simulink model "SIM_continuousFermenter"  (R2023b)
settings: Solver=VariableStepAuto  StartTime=0.0  StopTime=500  RelTol=1e-3
values from neighbouring files (symbols this model uses):
  Ts = 0.5    [MHE_compute2.m]
libraries: mpclib x1, SignalEditorBlockLib x1
settings Model: Creator=akeebismail  LastModifiedBy=akeebismail

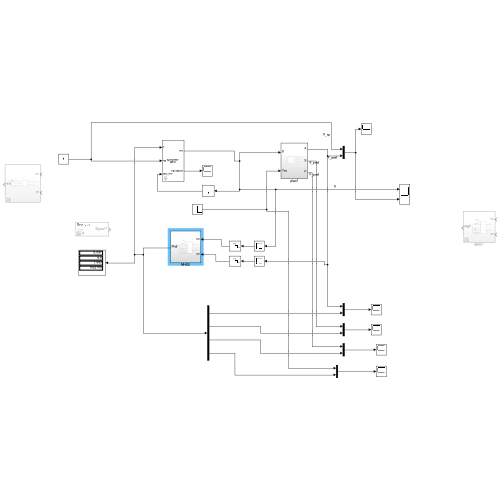
[thumbnail: Simulink's stored preview of the top-level diagram]
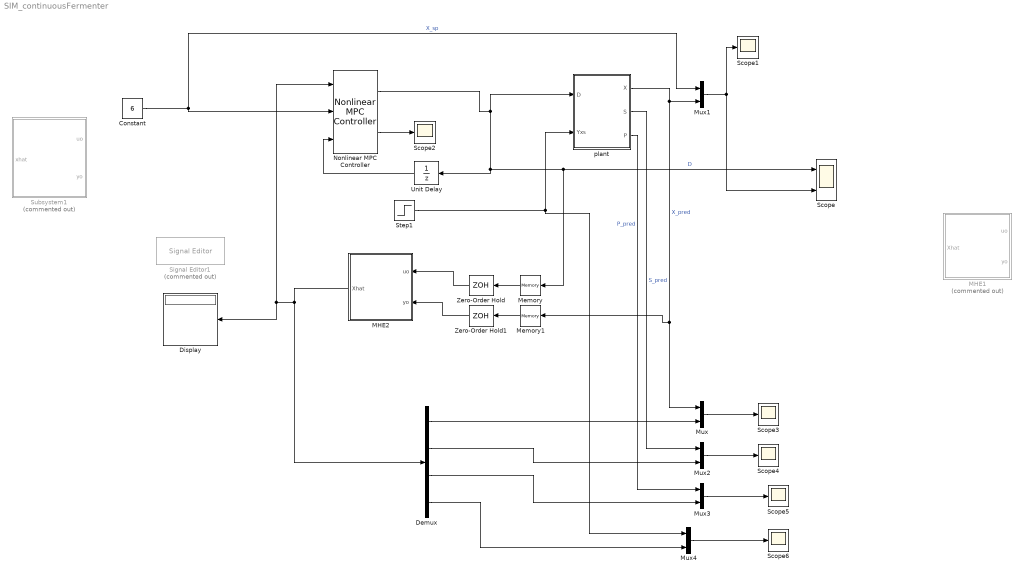
== system SIM_continuousFermenter ==
  Constant : Constant  Value=6
  Demux : Demux
  Display : Display
  MHE1 : Subsystem  Commented=on
  MHE2 : Subsystem
  Memory : Memory  InitialCondition=0.202
  Memory1 : Memory  InitialCondition=6
  Mux{,1..4} (5 alike) : Mux  Inputs=2
  Nonlinear MPC Controller : mpclib/Nonlinear MPC Controller  nlmpcobj=nlobj  UseObjectTs=on  UseMEX=off  md_enabled=off  mvtarget_enabled=off  param_enabled=off  cost_enabled=off  mvseq_enabled=off  stateseq_enabled=off  ovseq_enabled=off  slack_enabled=off  status_enabled=on  ov_min=off  ov_max=off  mv_min=off  mv_max=off  mvrate_min=off  mvrate_max=off  state_min=off  state_max=off  ov_weight=off  mv_weight=off  mvrate_weight=off  ecr_weight=off  nlp_initialize=off
  Scope : Scope  NumInputPorts=2
  Scope{1..6} (6 alike) : Scope
  Signal Editor1 : SignalEditorBlockLib/Signal Editor  Commented=on  FileName=Yxs.mat  ActiveScenario=Scenario  ActiveSignal=Signal 1  IsBus=off  OutputBusObjectStr=Bus: BusObject  SampleTime=Ts  Interpolate=off  ZeroCross=off  OutputAfterFinalValue=Setting to zero  Unit=inherit  PreserveSignalName=on  ApplySigPropsToAllScenarios=on  ApplySigPropsToAllSignals=off
  Step1 : Step  Time=200  Before=0.4  After=0.35  SampleTime=0
  Subsystem1 : Subsystem  Commented=on
  Unit Delay : UnitDelay  InitialCondition=0.202  SampleTime=Ts  HasFrameUpgradeWarning=on
  Zero-Order Hold : ZeroOrderHold  SampleTime=Ts
  Zero-Order Hold1 : ZeroOrderHold  SampleTime=Ts
  plant : Subsystem
  wires:
  Nonlinear MPC Controller/1 -> Memory/1, Scope/1, Unit Delay/1, plant/1(D)  "D"
  Constant/1 -> Nonlinear MPC Controller/2, Mux1/1  "X_sp"
  Nonlinear MPC Controller/2 -> Scope2/1
  plant/1(X) -> Mux/1, Memory1/1, Mux1/2  "X_pred"
  Unit Delay/1 -> Nonlinear MPC Controller/3
  Mux1/1 -> Scope/2, Scope1/1
  Zero-Order Hold/1 -> MHE2/1(uo)
  Zero-Order Hold1/1 -> MHE2/2(yo)
  Memory/1 -> Zero-Order Hold/1
  Memory1/1 -> Zero-Order Hold1/1
  MHE2/1(Xhat) -> Demux/1, Nonlinear MPC Controller/1, Display/1
  Demux/1 -> Mux/2
  Demux/2 -> Mux2/2
  Demux/3 -> Mux3/2
  Demux/4 -> Mux4/2
  plant/2(S) -> Mux2/1  "S_pred"
  plant/3(P) -> Mux3/1  "P_pred"
  Step1/1 -> Mux4/1, plant/2(Yxs)
  Mux/1 -> Scope3/1
  Mux2/1 -> Scope4/1
  Mux3/1 -> Scope5/1
  Mux4/1 -> Scope6/1

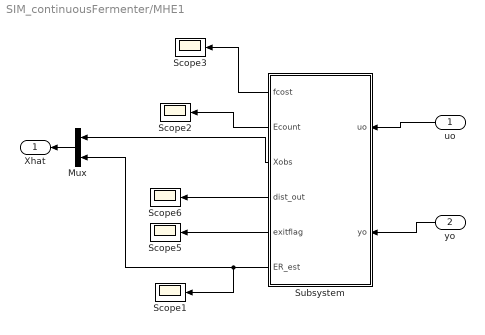
== system SIM_continuousFermenter/MHE1 ==
  uo : Inport
  yo : Inport  Port=2
  Mux : Mux  Inputs=2
  Scope{1..3,5..6} (5 alike) : Scope
  Subsystem : Subsystem
  Xhat : Outport
  wires:
  uo/1 -> Subsystem/1(uo)
  yo/1 -> Subsystem/2(yo)
  Subsystem/1(fcost) -> Scope3/1
  Subsystem/2(Ecount) -> Scope2/1
  Subsystem/6(ER_est) -> Mux/2, Scope1/1
  Subsystem/5(exitflag) -> Scope5/1
  Subsystem/4(dist_out) -> Scope6/1
  Mux/1 -> Xhat/1
  Subsystem/3(Xobs) -> Mux/1

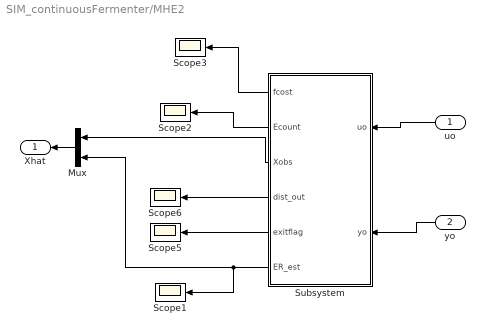
== system SIM_continuousFermenter/MHE2 ==
  uo : Inport
  yo : Inport  Port=2
  Mux : Mux  Inputs=2
  Scope{1..3,5..6} (5 alike) : Scope
  Subsystem : Subsystem
  Xhat : Outport
  wires:
  Subsystem/3(Xobs) -> Mux/1
  Mux/1 -> Xhat/1
  Subsystem/4(dist_out) -> Scope6/1
  Subsystem/5(exitflag) -> Scope5/1
  Subsystem/6(ER_est) -> Scope1/1, Mux/2
  Subsystem/2(Ecount) -> Scope2/1
  Subsystem/1(fcost) -> Scope3/1
  yo/1 -> Subsystem/2(yo)
  uo/1 -> Subsystem/1(uo)

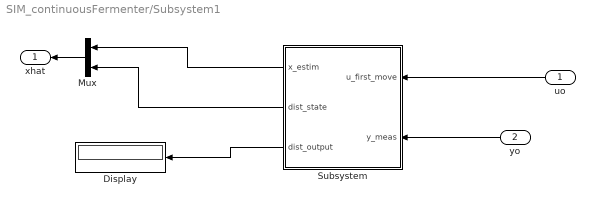
== system SIM_continuousFermenter/Subsystem1 ==
  uo : Inport
  yo : Inport  Port=2
  Display : Display
  Mux : Mux  Inputs=2
  Subsystem : Subsystem
  xhat : Outport
  wires:
  Mux/1 -> xhat/1
  yo/1 -> Subsystem/2(y_meas)
  uo/1 -> Subsystem/1(u_first_move)
  Subsystem/3(dist_output) -> Display/1
  Subsystem/2(dist_state) -> Mux/2
  Subsystem/1(x_estim) -> Mux/1

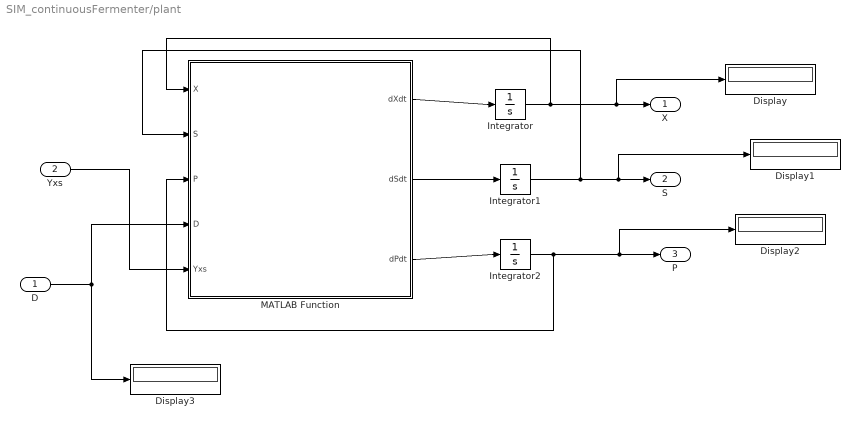
== system SIM_continuousFermenter/plant ==
  D : Inport
  Yxs : Inport  Port=2
  Display{,1..3} (4 alike) : Display
  Integrator : Integrator  InitialCondition=6
  Integrator1 : Integrator  InitialCondition=5
  Integrator2 : Integrator  InitialCondition=19.14
  MATLAB Function : MATLAB Function  TreatAsAtomicUnit=on
  X : Outport
  S : Outport  Port=2
  P : Outport  Port=3
  wires:
  MATLAB Function/1(dXdt) -> Integrator/1
  MATLAB Function/3(dPdt) -> Integrator2/1
  MATLAB Function/2(dSdt) -> Integrator1/1
  D/1 -> Display3/1, MATLAB Function/4(D)
  Integrator/1 -> Display/1, X/1, MATLAB Function/1(X)
  Integrator2/1 -> Display2/1, P/1, MATLAB Function/3(P)
  Integrator1/1 -> Display1/1, S/1, MATLAB Function/2(S)
  Yxs/1 -> MATLAB Function/5(Yxs)

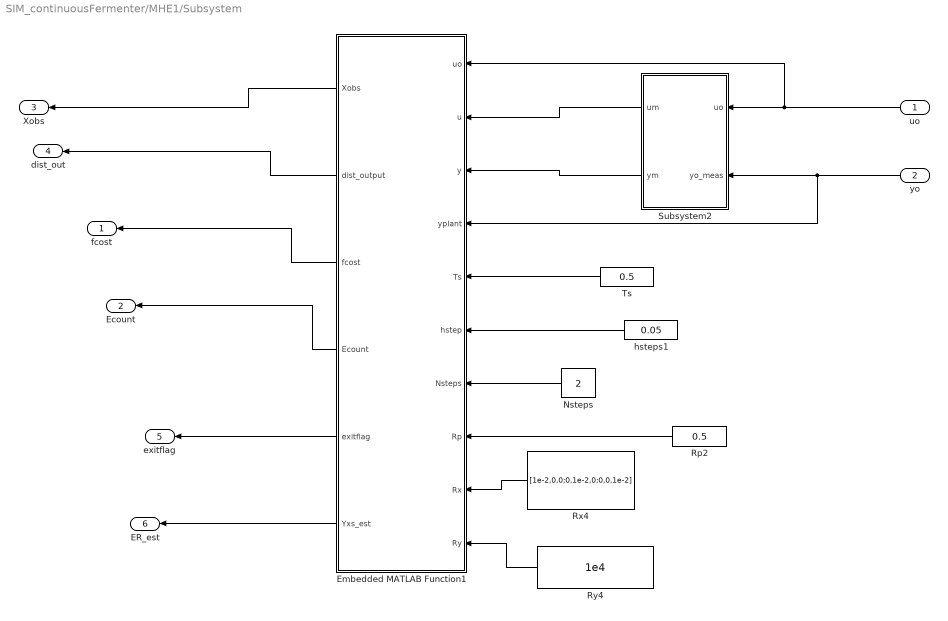
== system SIM_continuousFermenter/MHE1/Subsystem ==
  uo : Inport
  yo : Inport  Port=2
  Embedded MATLAB Function1 : MATLAB Function  TreatAsAtomicUnit=on
  Nsteps : Constant  Value=2
  Rp2 : Constant  Value=0.5
  Rx4 : Constant  Value=[1e-2,0,0;0,1e-2,0;0,0,1e-2]
  Ry4 : Constant  Value=1e4
  Subsystem2 : Subsystem
  Ts : Constant  Value=0.5
  hsteps1 : Constant  Value=0.05
  fcost : Outport  VectorParamsAs1DForOutWhenUnconnected=off
  Ecount : Outport  Port=2  VectorParamsAs1DForOutWhenUnconnected=off
  Xobs : Outport  Port=3  VectorParamsAs1DForOutWhenUnconnected=off
  dist_out : Outport  Port=4  VectorParamsAs1DForOutWhenUnconnected=off
  exitflag : Outport  Port=5  VectorParamsAs1DForOutWhenUnconnected=off
  ER_est : Outport  Port=6  VectorParamsAs1DForOutWhenUnconnected=off
  wires:
  Subsystem2/1(um) -> Embedded MATLAB Function1/2(u)
  Subsystem2/2(ym) -> Embedded MATLAB Function1/3(y)
  yo/1 -> Embedded MATLAB Function1/4(yplant), Subsystem2/2(yo_meas)
  uo/1 -> Embedded MATLAB Function1/1(uo), Subsystem2/1(uo)
  Nsteps/1 -> Embedded MATLAB Function1/7(Nsteps)
  hsteps1/1 -> Embedded MATLAB Function1/6(hstep)
  Embedded MATLAB Function1/3(fcost) -> fcost/1
  Embedded MATLAB Function1/4(Ecount) -> Ecount/1
  Rp2/1 -> Embedded MATLAB Function1/8(Rp)
  Rx4/1 -> Embedded MATLAB Function1/9(Rx)
  Ry4/1 -> Embedded MATLAB Function1/10(Ry)
  Embedded MATLAB Function1/1(Xobs) -> Xobs/1
  Embedded MATLAB Function1/2(dist_output) -> dist_out/1
  Embedded MATLAB Function1/5(exitflag) -> exitflag/1
  Embedded MATLAB Function1/6(Yxs_est) -> ER_est/1
  Ts/1 -> Embedded MATLAB Function1/5(Ts)

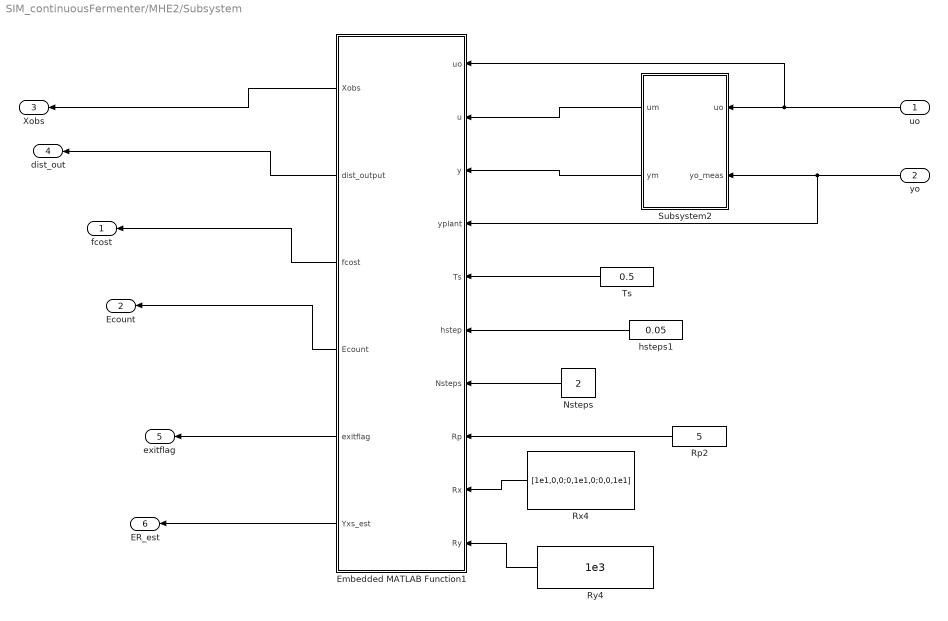
== system SIM_continuousFermenter/MHE2/Subsystem ==
  uo : Inport
  yo : Inport  Port=2
  Embedded MATLAB Function1 : MATLAB Function  TreatAsAtomicUnit=on
  Nsteps : Constant  Value=2
  Rp2 : Constant  Value=5
  Rx4 : Constant  Value=[1e1,0,0;0,1e1,0;0,0,1e1]
  Ry4 : Constant  Value=1e3
  Subsystem2 : Subsystem
  Ts : Constant  Value=0.5
  hsteps1 : Constant  Value=0.05
  fcost : Outport  VectorParamsAs1DForOutWhenUnconnected=off
  Ecount : Outport  Port=2  VectorParamsAs1DForOutWhenUnconnected=off
  Xobs : Outport  Port=3  VectorParamsAs1DForOutWhenUnconnected=off
  dist_out : Outport  Port=4  VectorParamsAs1DForOutWhenUnconnected=off
  exitflag : Outport  Port=5  VectorParamsAs1DForOutWhenUnconnected=off
  ER_est : Outport  Port=6  VectorParamsAs1DForOutWhenUnconnected=off
  wires:
  Ts/1 -> Embedded MATLAB Function1/5(Ts)
  Embedded MATLAB Function1/6(Yxs_est) -> ER_est/1
  Embedded MATLAB Function1/5(exitflag) -> exitflag/1
  Embedded MATLAB Function1/2(dist_output) -> dist_out/1
  Embedded MATLAB Function1/1(Xobs) -> Xobs/1
  Ry4/1 -> Embedded MATLAB Function1/10(Ry)
  Rx4/1 -> Embedded MATLAB Function1/9(Rx)
  Rp2/1 -> Embedded MATLAB Function1/8(Rp)
  Embedded MATLAB Function1/4(Ecount) -> Ecount/1
  Embedded MATLAB Function1/3(fcost) -> fcost/1
  hsteps1/1 -> Embedded MATLAB Function1/6(hstep)
  Nsteps/1 -> Embedded MATLAB Function1/7(Nsteps)
  uo/1 -> Subsystem2/1(uo), Embedded MATLAB Function1/1(uo)
  yo/1 -> Subsystem2/2(yo_meas), Embedded MATLAB Function1/4(yplant)
  Subsystem2/2(ym) -> Embedded MATLAB Function1/3(y)
  Subsystem2/1(um) -> Embedded MATLAB Function1/2(u)

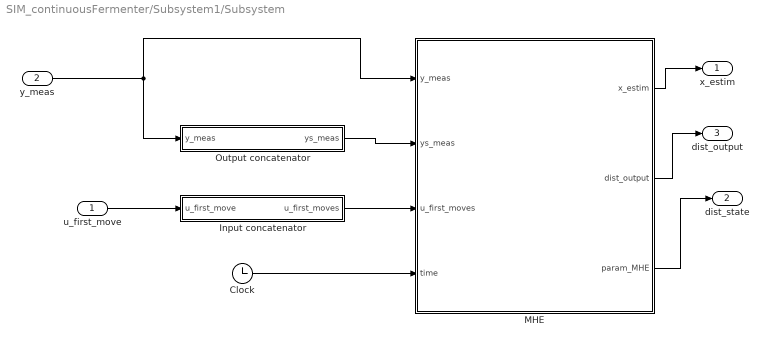
== system SIM_continuousFermenter/Subsystem1/Subsystem ==
  u_first_move : Inport  PortDimensions=[1,1]
  y_meas : Inport  Port=2  PortDimensions=[1,1]
  Clock : Clock
      settings: Decimation=20
  Input concatenator : Subsystem
  MHE : MATLAB Function  TreatAsAtomicUnit=on
  Output concatenator : Subsystem
  x_estim : Outport
  dist_state : Outport  Port=2
  dist_output : Outport  Port=3
  wires:
  Output concatenator/1(ys_meas) -> MHE/2(ys_meas)
  y_meas/1 -> Output concatenator/1(y_meas), MHE/1(y_meas)
  MHE/1(x_estim) -> x_estim/1
  u_first_move/1 -> Input concatenator/1(u_first_move)
  Clock/1 -> MHE/4(time)
  MHE/2(dist_output) -> dist_output/1
  MHE/3(param_MHE) -> dist_state/1
  Input concatenator/1(u_first_moves) -> MHE/3(u_first_moves)

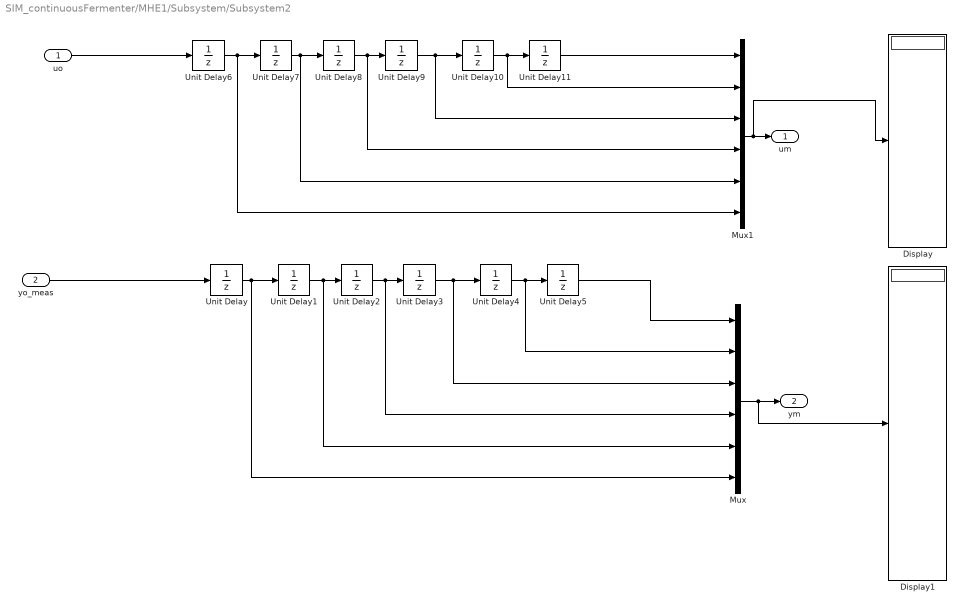
== system SIM_continuousFermenter/MHE1/Subsystem/Subsystem2 ==
  uo : Inport
  yo_meas : Inport  Port=2
  Display : Display
  Display1 : Display
  Mux : Mux  Inputs=6
  Mux1 : Mux  Inputs=6
  Unit Delay{,1..5} (6 alike) : UnitDelay  InitialCondition=6  SampleTime=Ts  HasFrameUpgradeWarning=on
  Unit Delay{6..11} (6 alike) : UnitDelay  InitialCondition=0.202  SampleTime=Ts  HasFrameUpgradeWarning=on
  um : Outport  VectorParamsAs1DForOutWhenUnconnected=off
  ym : Outport  Port=2  VectorParamsAs1DForOutWhenUnconnected=off
  wires:
  Unit Delay/1 -> Unit Delay1/1, Mux/6
  Unit Delay1/1 -> Unit Delay2/1, Mux/5
  Unit Delay2/1 -> Unit Delay3/1, Mux/4
  Unit Delay3/1 -> Unit Delay4/1, Mux/3
  Unit Delay4/1 -> Unit Delay5/1, Mux/2
  uo/1 -> Unit Delay6/1
  Unit Delay6/1 -> Mux1/6, Unit Delay7/1
  Unit Delay7/1 -> Mux1/5, Unit Delay8/1
  Unit Delay8/1 -> Mux1/4, Unit Delay9/1
  Unit Delay9/1 -> Mux1/3, Unit Delay10/1
  Unit Delay10/1 -> Unit Delay11/1, Mux1/2
  Mux/1 -> ym/1, Display1/1
  Mux1/1 -> um/1, Display/1
  Unit Delay11/1 -> Mux1/1
  Unit Delay5/1 -> Mux/1
  yo_meas/1 -> Unit Delay/1

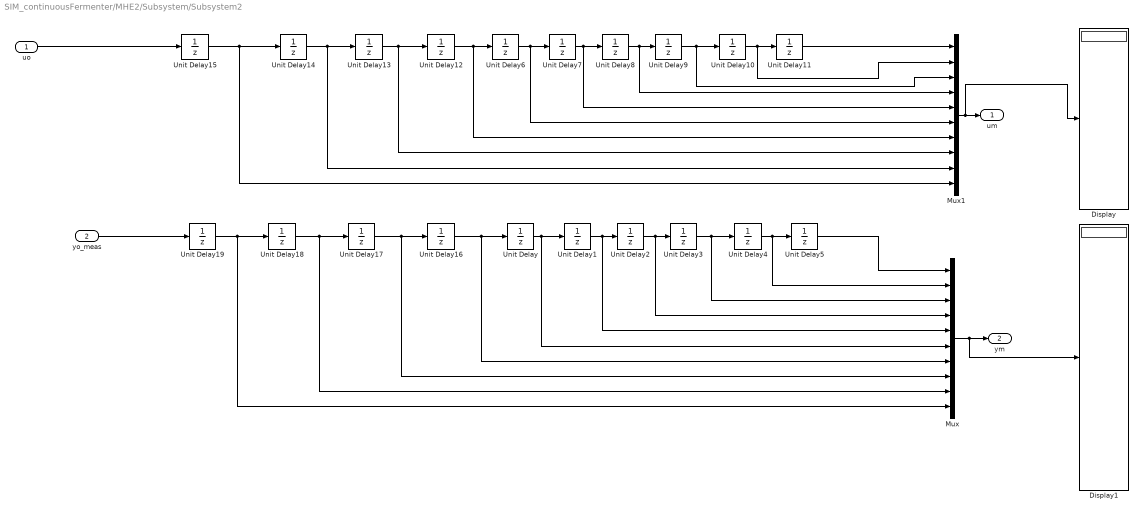
== system SIM_continuousFermenter/MHE2/Subsystem/Subsystem2 ==
  uo : Inport
  yo_meas : Inport  Port=2
  Display : Display
  Display1 : Display
  Mux : Mux  Inputs=10
  Mux1 : Mux  Inputs=10
  Unit Delay{,1..5,16..19} (10 alike) : UnitDelay  InitialCondition=6  SampleTime=Ts  HasFrameUpgradeWarning=on
  Unit Delay{6..15} (10 alike) : UnitDelay  InitialCondition=0.202  SampleTime=Ts  HasFrameUpgradeWarning=on
  um : Outport  VectorParamsAs1DForOutWhenUnconnected=off
  ym : Outport  Port=2  VectorParamsAs1DForOutWhenUnconnected=off
  wires:
  Unit Delay16/1 -> Mux/7, Unit Delay/1
  Unit Delay13/1 -> Mux1/8, Unit Delay12/1
  Unit Delay18/1 -> Mux/9, Unit Delay17/1
  Unit Delay2/1 -> Unit Delay3/1, Mux/4
  Mux1/1 -> um/1, Display/1
  Unit Delay17/1 -> Mux/8, Unit Delay16/1
  Unit Delay/1 -> Unit Delay1/1, Mux/6
  Unit Delay15/1 -> Mux1/10, Unit Delay14/1
  Unit Delay19/1 -> Mux/10, Unit Delay18/1
  Unit Delay8/1 -> Mux1/4, Unit Delay9/1
  yo_meas/1 -> Unit Delay19/1
  Unit Delay6/1 -> Mux1/6, Unit Delay7/1
  Unit Delay12/1 -> Mux1/7, Unit Delay6/1
  Unit Delay14/1 -> Mux1/9, Unit Delay13/1
  Unit Delay5/1 -> Mux/1
  Mux/1 -> ym/1, Display1/1
  Unit Delay3/1 -> Unit Delay4/1, Mux/3
  Unit Delay4/1 -> Unit Delay5/1, Mux/2
  Unit Delay9/1 -> Mux1/3, Unit Delay10/1
  Unit Delay10/1 -> Unit Delay11/1, Mux1/2
  Unit Delay7/1 -> Mux1/5, Unit Delay8/1
  Unit Delay1/1 -> Unit Delay2/1, Mux/5
  uo/1 -> Unit Delay15/1
  Unit Delay11/1 -> Mux1/1

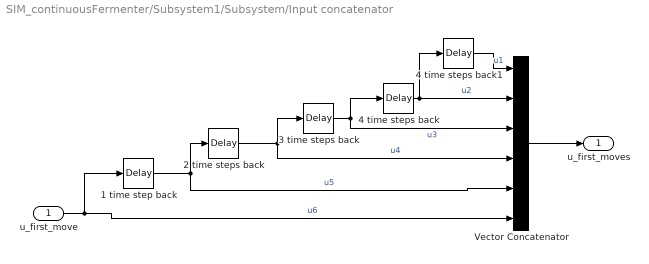
== system SIM_continuousFermenter/Subsystem1/Subsystem/Input concatenator ==
  u_first_move : Inport
  1 time step back : TransportDelay  DelayTime=Ts  InitialOutput=0.202
  2 time steps back : TransportDelay  DelayTime=Ts  InitialOutput=0.202
  3 time steps back : TransportDelay  DelayTime=Ts  InitialOutput=0.202
  4 time steps back : TransportDelay  DelayTime=Ts  InitialOutput=0.202
  4 time steps back1 : TransportDelay  DelayTime=Ts  InitialOutput=0.202
  Vector Concatenator : Concatenate  NumInputs=6  Mode=Multidimensional array
  u_first_moves : Outport  PortDimensions=[6,1]  VectorParamsAs1DForOutWhenUnconnected=off
  wires:
  4 time steps back1/1 -> Vector Concatenator/1  "u1"
  1 time step back/1 -> Vector Concatenator/5, 2 time steps back/1  "u5"
  2 time steps back/1 -> Vector Concatenator/4, 3 time steps back/1  "u4"
  3 time steps back/1 -> 4 time steps back/1, Vector Concatenator/3  "u3"
  4 time steps back/1 -> 4 time steps back1/1, Vector Concatenator/2  "u2"
  u_first_move/1 -> 1 time step back/1, Vector Concatenator/6  "u6"
  Vector Concatenator/1 -> u_first_moves/1

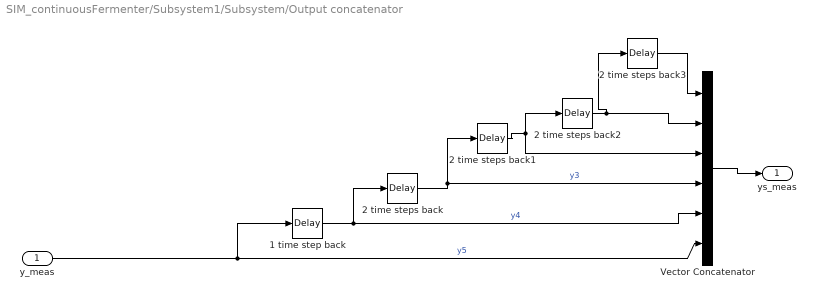
== system SIM_continuousFermenter/Subsystem1/Subsystem/Output concatenator ==
  y_meas : Inport
  1 time step back : TransportDelay  DelayTime=Ts  InitialOutput=6
  2 time steps back{,1..3} (4 alike) : TransportDelay  DelayTime=Ts  InitialOutput=6
  Vector Concatenator : Concatenate  NumInputs=6  Mode=Multidimensional array
  ys_meas : Outport  PortDimensions=[6,1]  VectorParamsAs1DForOutWhenUnconnected=off
  wires:
  2 time steps back3/1 -> Vector Concatenator/1
  y_meas/1 -> 1 time step back/1, Vector Concatenator/6  "y5"
  1 time step back/1 -> 2 time steps back/1, Vector Concatenator/5  "y4"
  2 time steps back/1 -> Vector Concatenator/4, 2 time steps back1/1  "y3"
  Vector Concatenator/1 -> ys_meas/1
  2 time steps back1/1 -> Vector Concatenator/3, 2 time steps back2/1
  2 time steps back2/1 -> Vector Concatenator/2, 2 time steps back3/1

== matlab function SIM_continuousFermenter/Subsystem1/Subsystem/MHE ==
  data: y_meas input; ys_meas input; x_estim output; u_first_moves input; time input; dist_output output; param_MHE output
function [x_estim,dist_output,param_MHE] = MHE_4_tanks(y_meas,ys_meas,u_first_moves,time)

coder.extrinsic('MHE_compute2');

N_MHE=6  ;
% Ts=2 ;


if time < 5
    
    x_estim =  [6;5;19.14]  ;
   % x_estim = [17;17;17];
    %x_estim = [5.898;1.8];
    param_MHE = 0.4;
    dist_output = 0;
else
    
    [x_estim,param_MHE,dist_output] = MHE_compute2(ys_meas,u_first_moves,N_MHE,y_meas);
    %Note that our horizon must be constant here. It is chosen as 5.
end

end

== matlab function SIM_continuousFermenter/plant/MATLAB Function ==
  data: X input; dXdt output; S input; P input; D input; dSdt output; dPdt output; Yxs input
function [dXdt,dSdt,dPdt] = continuous_fermenter(X,S,P,D,Yxs)

values = {22,1.2,50,20,2.2,0.2,0.48};

[Ki,Km,Pm,Sf,alpha,beta,miu_m] = values{:};


miu = (miu_m * (1 - (P/Pm))) * S / (Km + S + (S^2 / Ki))  ;

dXdt = -D * X + miu * X     ;

dSdt = D * (Sf - S) - (1/Yxs) * miu * X   ;

dPdt = -D * P + (alpha * miu + beta) * X   ;

end

== matlab function SIM_continuousFermenter/MHE2/Subsystem/Embedded MATLAB Function1 ==
  data: uo input; Xobs output size=[3,1]; dist_output output size=[1,1]; u input; y input; yplant input; Ts input; hstep input; Nsteps input; Rp input; fcost output size=[1,1]; Rx input; Ry input; Ecount output size=[1,1]; exitflag output size=[1,1]; Yxs_est output size=[1,1]
function [Xobs,dist_output,fcost,Ecount,exitflag,Yxs_est] =MHE(uo,u,y,yplant,Ts,hstep,Nsteps,Rp,Rx,Ry)

%#codegen
coder.extrinsic('MHE_compute','clear_var');

um=[u(1),u(2),u(3),u(4),u(5),u(6),u(7),u(8),u(9),u(10)] ;
 

ymeas=[y(1),y(2),y(3),y(4),y(5),y(6),y(7),y(8),y(9),y(10)] ;


    
   

% SAMPLING TIME FOR DISCRETIZATION
%hstep=1; %sampling time of 10 is with less interation while 5 is smoother but higher interaction
%Nsteps=1 ;% Nsteps=10 ; % Nsteps=20 ;


d_initial=[6;5;19.14;0.4]   ;
%d_MIN_colvector =[0;0;100]  ;
d_MIN_colvector =[0;0;0;0]  ;
d_MAX_colvector =[20;60;60;1]  ;
%%%%%%%%%%%%%%%%%%%%%%%%%%%%%%%%%%%%%%%
%Initializing variables
fcost=inf  ;
Xobs=[0;0;0]  ;
%d_opt=[0;0]  ;
dist_output = [0]  ;
Yxs_est=[0]  ;
Ecount=0  ;
exitflag=2   ;

% [Xobs,dist_output,fcost,Ecount,exitflag]=MHE_compute(uo,um,ymeas,yplant...
%                                         ,hstep,Nsteps,Nmhe,Rp,Rx,Ry...
%                                         ,p_initial, p_MIN_colvector,p_MAX_colvector)
[Xobs,dist_output,Yxs_est,fcost,Ecount,exitflag]=MHE_compute(uo,um,ymeas...
                                        ,yplant,Ts,hstep,Nsteps,Rp,Rx,Ry...
                                        ,d_initial, d_MIN_colvector,d_MAX_colvector);

== matlab function SIM_continuousFermenter/MHE1/Subsystem/Embedded MATLAB Function1 ==
  data: uo input; Xobs output size=[3,1]; dist_output output size=[1,1]; u input; y input; yplant input; Ts input; hstep input; Nsteps input; Rp input; fcost output size=[1,1]; Rx input; Ry input; Ecount output size=[1,1]; exitflag output size=[1,1]; Yxs_est output size=[1,1]
function [Xobs,dist_output,fcost,Ecount,exitflag,Yxs_est] =MHE(uo,u,y,yplant,Ts,hstep,Nsteps,Rp,Rx,Ry)

%#codegen
coder.extrinsic('MHE_compute','clear_var');

um=[u(1),u(2),u(3),u(4),u(5),u(6)] ;
 

ymeas=[y(1),y(2),y(3),y(4),y(5),y(6)] ;


    
   

% SAMPLING TIME FOR DISCRETIZATION
%hstep=1; %sampling time of 10 is with less interation while 5 is smoother but higher interaction
%Nsteps=1 ;% Nsteps=10 ; % Nsteps=20 ;


d_initial=[6;5;19.14;0.4]   ;
%d_MIN_colvector =[0;0;100]  ;
d_MIN_colvector =[0;0;0;0]  ;
d_MAX_colvector =[20;60;60;1]  ;
%%%%%%%%%%%%%%%%%%%%%%%%%%%%%%%%%%%%%%%
%Initializing variables
fcost=inf  ;
Xobs=[0;0;0]  ;
%d_opt=[0;0]  ;
dist_output = [0]  ;
Yxs_est=[0]  ;
Ecount=0  ;
exitflag=2   ;

% [Xobs,dist_output,fcost,Ecount,exitflag]=MHE_compute(uo,um,ymeas,yplant...
%                                         ,hstep,Nsteps,Nmhe,Rp,Rx,Ry...
%                                         ,p_initial, p_MIN_colvector,p_MAX_colvector)
[Xobs,dist_output,Yxs_est,fcost,Ecount,exitflag]=MHE_compute(uo,um,ymeas...
                                        ,yplant,Ts,hstep,Nsteps,Rp,Rx,Ry...
                                        ,d_initial, d_MIN_colvector,d_MAX_colvector);
